simulink model "JT9D_Model_Dyn"  (Simulink 8.5)
settings: Solver=ode4  StartTime=0.0  StopTime=30  FixedStep=0.04  RelTol=1e-3
values from neighbouring files (symbols this model uses):
  MWS = setup_Inputs(MWS)    [JT9D_setup_everything_Dyn.m]    (also in JT9D_setup_everything_Lin.m; JT9D_setup_everything_PWLinGen.m; JT9D_setup_everything_SS.m)
undefined symbols (not defined in the file or in its folder): stripchar_TMATS
libraries: Lib_Turbo_Duct_TMATS x5, Lib_Turbo_Compressor_TMATS x3, Lib_Solve_OuterLoopIntegrator_TMATS x2, Lib_Turbo_Shaft_TMATS x2, Lib_Turbo_TurbineNPSS_TMATS x2, Lib_Turbo_Nozzle_TMATS x2, Lib_Cntrl_SimplePIcontroller_TMATS x1, Lib_Solve_IterNRSolverJC_TMATS x1, Lib_Turbo_Burner_TMATS x1, Lib_Turbo_Inlet_TMATS x1, Lib_Turbo_Splitter_TMATS x1
settings Model: Creator=jwchapm2  LastModifiedBy=jwchapm2
settings DataIOCC: SignalLoggingSaveFormat=Dataset
settings DebuggingCC: SolverPrmCheckMsg=warning  FcnCallInpInsideContextMsg=EnableAllAsError
settings GRTTargetCC: CombineOutputUpdateFcns=on  GRTInterface=off

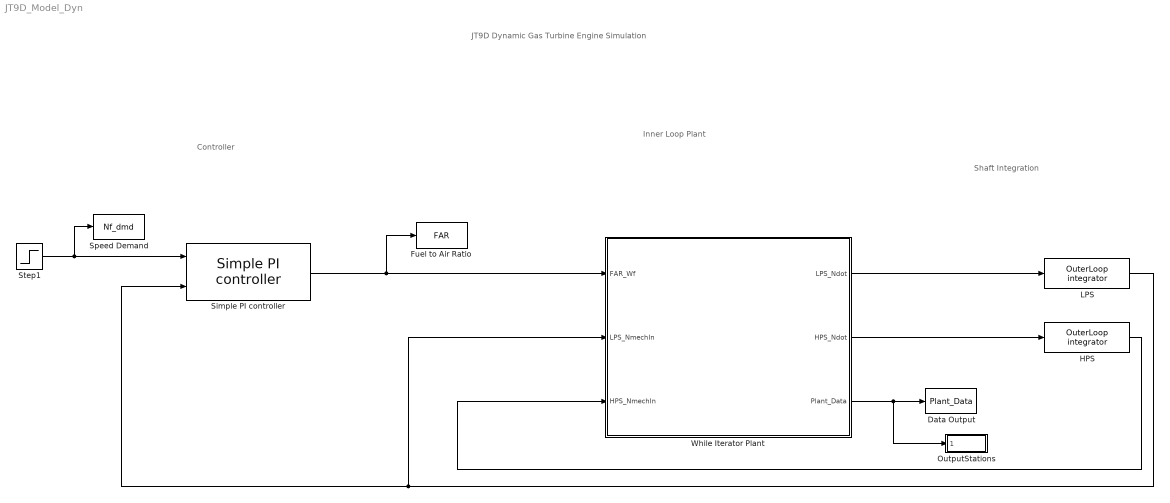
== system JT9D_Model_Dyn ==
  note: JT9D Dynamic Gas Turbine Engine Simulation
  note: Controller
  note: Inner Loop Plant
  note: Shaft Integration
  Data Output : ToWorkspace  VariableName=Plant_Data  SaveFormat=Timeseries  SampleTime=-1
  Fuel to Air Ratio : ToWorkspace  VariableName=FAR  SaveFormat=Timeseries  SampleTime=-1
  HPS : Lib_Solve_OuterLoopIntegrator_TMATS/OuterLoop integrator  OL_IC_M=MWS.Input.HP_Shaft
  LPS : Lib_Solve_OuterLoopIntegrator_TMATS/OuterLoop integrator  OL_IC_M=MWS.Input.LP_Shaft
  OutputStations : Subsystem
  Simple PI controller : Lib_Cntrl_SimplePIcontroller_TMATS/Simple PI controller  Kp_M=0.000008  Ki_M=0.00001  PI_IC_M=MWS.Input.FARin
  Speed Demand : ToWorkspace  VariableName=Nf_dmd  SaveFormat=Timeseries  SampleTime=-1
  Step1 : Step  Time=15  Before=MWS.Input.LP_Shaft  After=MWS.Input.LP_Shaft -200  SampleTime=0
  While Iterator Plant : Subsystem  TreatAsAtomicUnit=on
  wires:
  While Iterator Plant/1(LPS_Ndot) -> LPS/1
  While Iterator Plant/2(HPS_Ndot) -> HPS/1
  LPS/1 -> Simple PI controller/2, While Iterator Plant/2(LPS_NmechIn)
  HPS/1 -> While Iterator Plant/3(HPS_NmechIn)
  Simple PI controller/1 -> Fuel to Air Ratio/1, While Iterator Plant/1(FAR_Wf)
  Step1/1 -> Speed Demand/1, Simple PI controller/1
  While Iterator Plant/3(Plant_Data) -> OutputStations/1(DataBus), Data Output/1

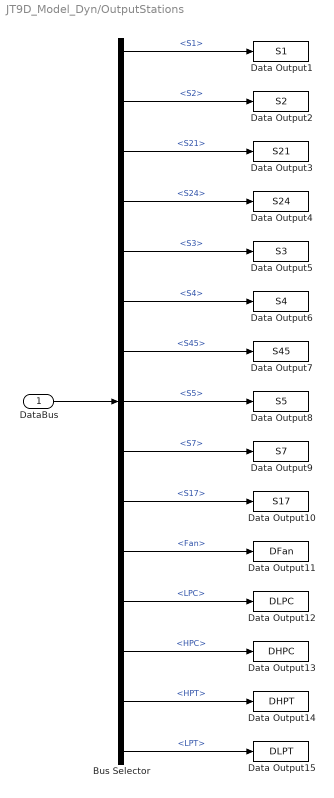
== system JT9D_Model_Dyn/OutputStations ==
  DataBus : Inport
  Bus Selector : BusSelector  OutputSignals=StationData.S1,StationData.S2,StationData.S21,StationData.S24,StationData.S3,StationData.S4,StationData.S45,StationData.S5,StationData.S7,StationData.S17,Data.Fan,Data.LPC,Data.HPC,Data.HPT,Data.LPT
  Data Output1 : ToWorkspace  VariableName=S1  SaveFormat=Timeseries  SampleTime=-1
  Data Output10 : ToWorkspace  VariableName=S17  SaveFormat=Timeseries  SampleTime=-1
  Data Output11 : ToWorkspace  VariableName=DFan  SaveFormat=Timeseries  SampleTime=-1
  Data Output12 : ToWorkspace  VariableName=DLPC  SaveFormat=Timeseries  SampleTime=-1
  Data Output13 : ToWorkspace  VariableName=DHPC  SaveFormat=Timeseries  SampleTime=-1
  Data Output14 : ToWorkspace  VariableName=DHPT  SaveFormat=Timeseries  SampleTime=-1
  Data Output15 : ToWorkspace  VariableName=DLPT  SaveFormat=Timeseries  SampleTime=-1
  Data Output2 : ToWorkspace  VariableName=S2  SaveFormat=Timeseries  SampleTime=-1
  Data Output3 : ToWorkspace  VariableName=S21  SaveFormat=Timeseries  SampleTime=-1
  Data Output4 : ToWorkspace  VariableName=S24  SaveFormat=Timeseries  SampleTime=-1
  Data Output5 : ToWorkspace  VariableName=S3  SaveFormat=Timeseries  SampleTime=-1
  Data Output6 : ToWorkspace  VariableName=S4  SaveFormat=Timeseries  SampleTime=-1
  Data Output7 : ToWorkspace  VariableName=S45  SaveFormat=Timeseries  SampleTime=-1
  Data Output8 : ToWorkspace  VariableName=S5  SaveFormat=Timeseries  SampleTime=-1
  Data Output9 : ToWorkspace  VariableName=S7  SaveFormat=Timeseries  SampleTime=-1
  wires:
  DataBus/1 -> Bus Selector/1
  Bus Selector/1 -> Data Output1/1  "<S1>"
  Bus Selector/2 -> Data Output2/1  "<S2>"
  Bus Selector/3 -> Data Output3/1  "<S21>"
  Bus Selector/4 -> Data Output4/1  "<S24>"
  Bus Selector/5 -> Data Output5/1  "<S3>"
  Bus Selector/6 -> Data Output6/1  "<S4>"
  Bus Selector/7 -> Data Output7/1  "<S45>"
  Bus Selector/8 -> Data Output8/1  "<S5>"
  Bus Selector/9 -> Data Output9/1  "<S7>"
  Bus Selector/10 -> Data Output10/1  "<S17>"
  Bus Selector/11 -> Data Output11/1  "<Fan>"
  Bus Selector/12 -> Data Output12/1  "<LPC>"
  Bus Selector/13 -> Data Output13/1  "<HPC>"
  Bus Selector/14 -> Data Output14/1  "<HPT>"
  Bus Selector/15 -> Data Output15/1  "<LPT>"

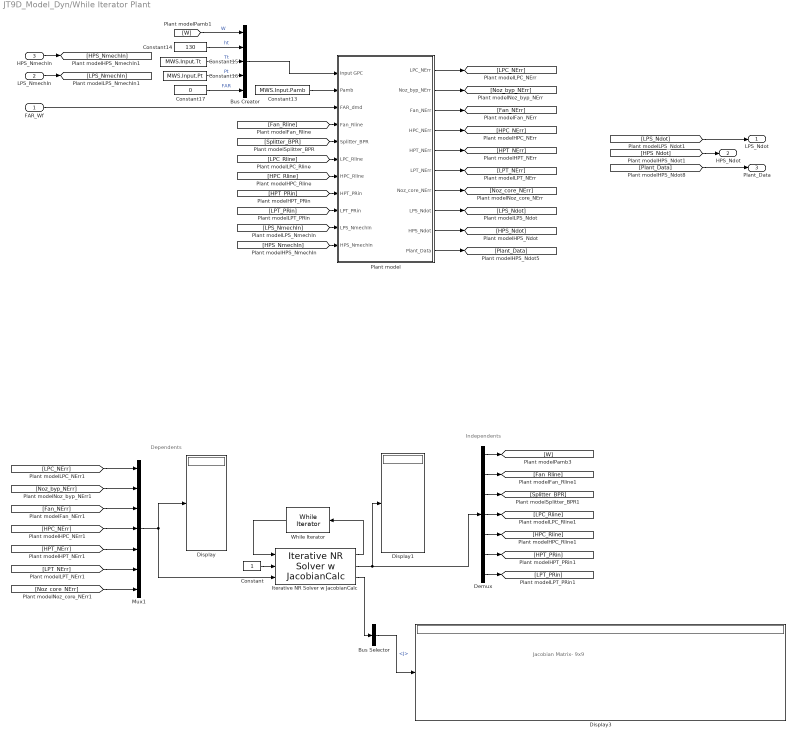
== system JT9D_Model_Dyn/While Iterator Plant ==
  note: Jacobian Matrix- 9x9
  note: Dependents
  note: Independents
  FAR_Wf : Inport
  LPS_NmechIn : Inport  Port=2
  HPS_NmechIn : Inport  Port=3
  Bus Creator : BusCreator  Inputs=5
  Bus Selector : BusSelector  OutputSignals=J
  Constant : Constant
  Constant13 : Constant  Value=MWS.Input.Pamb
  Constant14 : Constant  Value=130
  Constant15 : Constant  Value=MWS.Input.Tt
  Constant16 : Constant  Value=MWS.Input.Pt
  Constant17 : Constant  Value=0
  Demux : Demux  Outputs=7
  Display : Display
  Display1 : Display
  Display3 : Display
  Iterative NR Solver w JacobianCalc : Lib_Solve_IterNRSolverJC_TMATS/Iterative NR Solver w JacobianCalc  SJac_Per_M=[0.05 0.05 0.05 0.05 0.05 0.05 0.05]  SNR_IC_M=MWS.Input.NRICDyn  SNR_DX_M=5  SNR_Mx_M=100000  SNR_Mn_M=0.0001  SJacobianAttempts_M=20  Cond_Limits_M=0.0001
  Mux1 : Mux  Inputs=7
  Plant model : Subsystem
  While Iterator : WhileIterator  WhileBlockType=do-while  ShowIterationPort=on
  LPS_Ndot : Outport
  HPS_Ndot : Outport  Port=2
  Plant_Data : Outport  Port=3
  wires:
  [W] -> Bus Creator/1  "W"
  Bus Creator/1 -> Plant model/1(Input GPC)
  Constant17/1 -> Bus Creator/5  "FAR"
  Constant15/1 -> Bus Creator/3  "Tt"
  Constant16/1 -> Bus Creator/4  "Pt"
  Constant14/1 -> Bus Creator/2  "ht"
  Constant13/1 -> Plant model/2(Pamb)
  FAR_Wf/1 -> Plant model/3(FAR_dmd)
  [Fan_Rline] -> Plant model/4(Fan_Rline)
  [Splitter_BPR] -> Plant model/5(Splitter_BPR)
  [LPC_Rline] -> Plant model/6(LPC_Rline)
  [HPC_Rline] -> Plant model/7(HPC_Rline)
  [HPT_PRin] -> Plant model/8(HPT_PRin)
  [LPT_PRin] -> Plant model/9(LPT_PRin)
  [LPS_NmechIn] -> Plant model/10(LPS_NmechIn)
  [HPS_NmechIn] -> Plant model/11(HPS_NmechIn)
  Plant model/1(LPC_NErr) -> [LPC_NErr]
  Plant model/2(Noz_byp_NErr) -> [Noz_byp_NErr]
  Plant model/3(Fan_NErr) -> [Fan_NErr]
  Plant model/4(HPC_NErr) -> [HPC_NErr]
  Plant model/5(HPT_NErr) -> [HPT_NErr]
  Plant model/6(LPT_NErr) -> [LPT_NErr]
  Plant model/7(Noz_core_NErr) -> [Noz_core_NErr]
  Plant model/8(LPS_Ndot) -> [LPS_Ndot]
  Plant model/9(HPS_Ndot) -> [HPS_Ndot]
  Demux/1 -> [W]
  Demux/7 -> [LPT_PRin]
  Demux/5 -> [HPC_Rline]
  Demux/6 -> [HPT_PRin]
  Demux/4 -> [LPC_Rline]
  Demux/2 -> [Fan_Rline]
  Demux/3 -> [Splitter_BPR]
  [Fan_NErr] -> Mux1/3
  [HPC_NErr] -> Mux1/4
  [Noz_byp_NErr] -> Mux1/2
  [HPT_NErr] -> Mux1/5
  [LPC_NErr] -> Mux1/1
  [LPT_NErr] -> Mux1/6
  [Noz_core_NErr] -> Mux1/7
  Iterative NR Solver w JacobianCalc/3 -> Bus Selector/1
  Mux1/1 -> Iterative NR Solver w JacobianCalc/3, Display/1
  Bus Selector/1 -> Display3/1  "<J>"
  Iterative NR Solver w JacobianCalc/2 -> Demux/1, Display1/1
  Iterative NR Solver w JacobianCalc/1 -> While Iterator/1
  HPS_NmechIn/1 -> [HPS_NmechIn]
  LPS_NmechIn/1 -> [LPS_NmechIn]
  [LPS_Ndot] -> LPS_Ndot/1
  [HPS_Ndot] -> HPS_Ndot/1
  Plant model/10(Plant_Data) -> [Plant_Data]
  [Plant_Data] -> Plant_Data/1
  Constant/1 -> Iterative NR Solver w JacobianCalc/2
  While Iterator/1 -> Iterative NR Solver w JacobianCalc/1

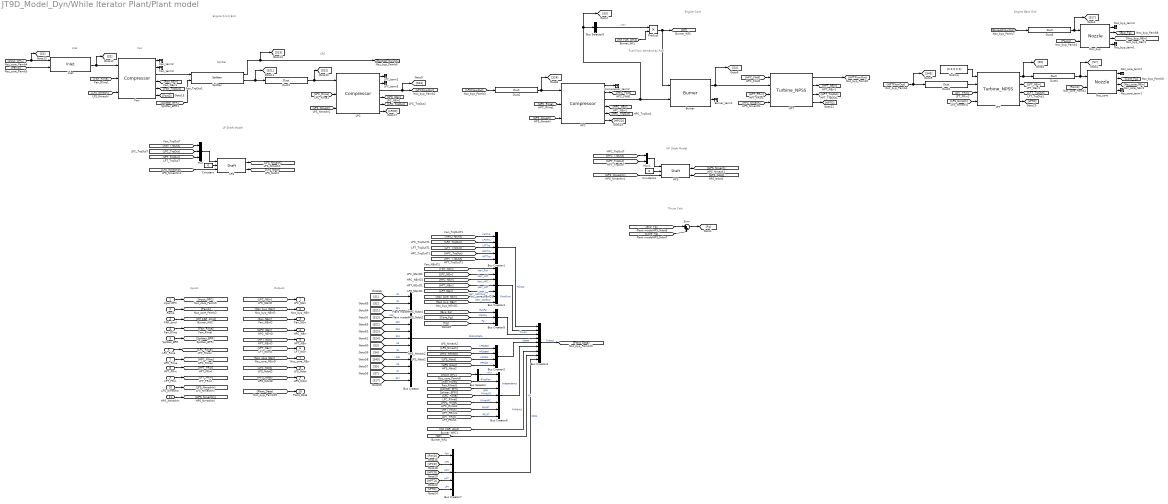
== system JT9D_Model_Dyn/While Iterator Plant/Plant model ==
  note: LP Shaft Model
  note: Inputs
  note: Outputs
  note: Engine Core
  note: HP Shaft Model
  note: Engine Back End
  note: Engine Front End
  note: Fuel Flow demand as FAR
  note: Inlet
  note: Fan
  note: Splitter
  note: LPC
  note: Thrust Calc
  Input GPC : Inport
  Pamb : Inport  Port=2
  FAR_dmd : Inport  Port=3
  Fan_Rline : Inport  Port=4
  Splitter_BPR : Inport  Port=5
  LPC_Rline : Inport  Port=6
  HPC_Rline : Inport  Port=7
  HPT_PRin : Inport  Port=8
  LPT_PRin : Inport  Port=9
  LPS_NmechIn : Inport  Port=10
  HPS_NmechIn : Inport  Port=11
  Burner : Lib_Turbo_Burner_TMATS/Burner  LHVEn_M=on  LHV_M=18400  Eff_M=0.994  hFuel_M=-1200  dPnormBurner_M=MWS.Burn.dP
  Burner_term1 : Terminator
  Bus Creator : BusCreator  Inputs=13
  Bus Creator1 : BusCreator  Inputs=5
  Bus Creator2 : BusCreator
  Bus Creator3 : BusCreator  Inputs=9
  Bus Creator4 : BusCreator  Inputs=7
  Bus Creator5 : BusCreator  Inputs=3
  Bus Creator6 : BusCreator  Inputs=7
  Bus Creator7 : BusCreator  Inputs=5
  Bus Selector : BusSelector  OutputSignals=W
  Bus Selector5 : BusSelector  OutputSignals=W
  Compressor_term2 : Terminator
  Constant : Constant  Value=0
  Constant1 : Constant  Value=0
  Duct1 : Lib_Turbo_Duct_TMATS/Duct  dP_M=MWS.Duct.dP1
  Duct2 : Lib_Turbo_Duct_TMATS/Duct  dP_M=MWS.Duct.dP2
  Duct3 : Lib_Turbo_Duct_TMATS/Duct  dP_M=MWS.Duct.dP3
  Duct4 : Lib_Turbo_Duct_TMATS/Duct  dP_M=MWS.Duct.dP4
  Duct5 : Lib_Turbo_Duct_TMATS/Duct  dP_M=MWS.Duct.dP5
  Fan : Lib_Turbo_Compressor_TMATS/Compressor  X_C_RlineVec_M=MWS.FAN.RlineVec  Z_C_AlphaVec_M=1  Y_C_Map_NcVec_M=MWS.FAN.NcVec  T_C_Map_WcArray_M=MWS.FAN.WcArray  T_C_Map_PRArray_M=MWS.FAN.PRArray  T_C_Map_EffArray_M=MWS.FAN.EffArray  s_C_Nc_M=MWS.FAN.s_Nc  s_C_Wc_M=MWS.FAN.s_Wc  s_C_PR_M=MWS.FAN.s_PR  s_C_Eff_M=MWS.FAN.s_eff  SL_M=off  Scale_M=none  CBLDEN_M=off  C_CBD_M=0  C_CBFht_M=0.5  C_CBFPt_M=0.5  FBLDEN_M=off  C_FBD_M=0  C_BFht_M=0.5  C_BFPt_M=0.5  DefSMEn_M=on  SRline_M=1  X_C_Map_WcSurgeVec_M=[0 200]  T_C_Map_PRSurgeVec_M=[30 30]  iDesign_M=MWS.iDes  NcDes_M=1  EffDes_M=0.8675  PRDes_M=1.645  RlineDes_M=2.3706  FVar_M=strcat('iDes_',stripchar_TMATS(gcb),'.bin')  BlkNm_M=double(gcb)  HP_M=off
  Fan_term2 : Terminator
  Fan_term3 : Terminator
  HPC : Lib_Turbo_Compressor_TMATS/Compressor  X_C_RlineVec_M=MWS.HPC.RlineVec  Z_C_AlphaVec_M=1  Y_C_Map_NcVec_M=MWS.HPC.NcVec  T_C_Map_WcArray_M=MWS.HPC.WcArray  T_C_Map_PRArray_M=MWS.HPC.PRArray  T_C_Map_EffArray_M=MWS.HPC.EffArray  s_C_Nc_M=MWS.HPC.s_Nc  s_C_Wc_M=MWS.HPC.s_Wc  s_C_PR_M=MWS.HPC.s_PR  s_C_Eff_M=MWS.HPC.s_eff  SL_M=off  Scale_M=none  CBLDEN_M=off  C_CBD_M=0  C_CBFht_M=0.5  C_CBFPt_M=0.5  FBLDEN_M=on  C_FBD_M=MWS.HPC.Fbld  C_BFht_M=MWS.HPC.Fblde  C_BFPt_M=MWS.HPC.Fbldp  DefSMEn_M=on  SRline_M=1  X_C_Map_WcSurgeVec_M=[0 200]  T_C_Map_PRSurgeVec_M=[30 30]  iDesign_M=MWS.iDes  NcDes_M=0.995  EffDes_M=.8651  PRDes_M=5.609  RlineDes_M=2.0424  FVar_M=strcat('iDes_',stripchar_TMATS(gcb),'.bin')  BlkNm_M=double(gcb)  HP_M=off
  HPS : Lib_Turbo_Shaft_TMATS/Shaft  Shaft_Inertia_M=MWS.Shaft.Iner_hp
  HPT : Lib_Turbo_TurbineNPSS_TMATS/Turbine_NPSS  X_T_Map_PRVec_M=MWS.HPT.PRVec  Y_T_Map_NcVec_M=MWS.HPT.NcVec  T_T_Map_WcArray_M=MWS.HPT.WcArray  T_T_Map_EffArray_M=MWS.HPT.EffArray  s_T_Nc_M=MWS.HPT.s_Nc  s_T_Wc_M=MWS.HPT.s_Wc  s_T_PR_M=MWS.HPT.s_PR  s_T_Eff_M=MWS.HPT.s_eff  ConfigNPSS_M=1  Scale_M=none  CFlwEn_M=on  T_CoolFlwPos_M=MWS.HPT.Cool  iDesign_M=MWS.iDes  NcDes_M=99.031  EffDes_M=.9133  PRDes_M=4.930  NDes_M=7390  FVar_M=strcat('iDes_',stripchar_TMATS(gcb),'.bin')  BlkNm_M=double(gcb)  HP_M=off
  Inlet : Lib_Turbo_Inlet_TMATS/Inlet  eRambase_M=MWS.Inlet.eRamBase  X_eRamVec_M=MWS.Inlet.eRamVec  T_eRamtbl_M=MWS.Inlet.eRamtbl
  LPC : Lib_Turbo_Compressor_TMATS/Compressor  X_C_RlineVec_M=MWS.LPC.RlineVec  Z_C_AlphaVec_M=1  Y_C_Map_NcVec_M=MWS.LPC.NcVec  T_C_Map_WcArray_M=MWS.LPC.WcArray  T_C_Map_PRArray_M=MWS.LPC.PRArray  T_C_Map_EffArray_M=MWS.LPC.EffArray  s_C_Nc_M=MWS.LPC.s_Nc  s_C_Wc_M=MWS.LPC.s_Wc  s_C_PR_M=MWS.LPC.s_PR  s_C_Eff_M=MWS.LPC.s_eff  SL_M=off  Scale_M=none  CBLDEN_M=off  C_CBD_M=0  C_CBFht_M=0.5  C_CBFPt_M=0.5  FBLDEN_M=off  C_FBD_M=0  C_BFht_M=0.5  C_BFPt_M=0.5  DefSMEn_M=on  SRline_M=1  X_C_Map_WcSurgeVec_M=[0 200]  T_C_Map_PRSurgeVec_M=[30 30]  iDesign_M=MWS.iDes  NcDes_M=0.993  EffDes_M=.8683  PRDes_M=2.488  RlineDes_M=1.7664  FVar_M=strcat('iDes_',stripchar_TMATS(gcb),'.bin')  BlkNm_M=double(gcb)  HP_M=off
  LPC_term2 : Terminator
  LPC_term3 : Terminator
  LPS : Lib_Turbo_Shaft_TMATS/Shaft  Shaft_Inertia_M=MWS.Shaft.Iner_lp
  LPT : Lib_Turbo_TurbineNPSS_TMATS/Turbine_NPSS  X_T_Map_PRVec_M=MWS.LPT.PRVec  Y_T_Map_NcVec_M=MWS.LPT.NcVec  T_T_Map_WcArray_M=MWS.LPT.WcArray  T_T_Map_EffArray_M=MWS.LPT.EffArray  s_T_Nc_M=MWS.LPT.s_Nc  s_T_Wc_M=MWS.LPT.s_Wc  s_T_PR_M=MWS.LPT.s_PR  s_T_Eff_M=MWS.LPT.s_eff  ConfigNPSS_M=1  Scale_M=none  CFlwEn_M=off  T_CoolFlwPos_M=0  iDesign_M=MWS.iDes  NcDes_M=105.038  EffDes_M=.9323  PRDes_M=6.420  NDes_M=3667.6  FVar_M=strcat('iDes_',stripchar_TMATS(gcb),'.bin')  BlkNm_M=double(gcb)  HP_M=off
  Mux : Mux  Inputs=3
  Mux1 : Mux  Inputs=2
  NoFlow : Constant  Value=[0 0 0 0 0]
  Noz_byp : Lib_Turbo_Nozzle_TMATS/Nozzle  SWType_M=Convergent  N_TArea_M=MWS.NozB.Ath  N_EArea_M=110.7  N_FL_M=0.00  X_N_TtVec2_M=[300 2000]  T_N_TGArray_M=[1 1]  X_N_PEQPaVec_M=[0 10000]  T_N_CdThArray_M=[1 1]  T_N_CvArray_M=MWS.NozB.CvArray  CfgEn_M=off  T_N_CfgArray_M=[1 1]  X_N_FARVec_M=[0; 0.0050; 0.0100; 0.0150; 0.0200; 0.0250; 0.0300]  T_N_RtArray_M="[0.0686;    0.0686;    0.0686;    0.0686;    0.0686;    0.0686;    0.0686]"  Y_N_TtVec_M=[300 2000]  T_N_MAP_gammaArray_M=[ 1.4 1.4 1.4 1.4 1.4 1.4 1.4; 1.4 1.4 1.4 1.4 1.4 1.4 1.4]  iDesign_M=MWS.iDes  WDes_M=562.61  FVar_M=strcat('iDes_',stripchar_TMATS(gcb),'.bin')
  Noz_byp_term1 : Terminator
  Noz_byp_term3 : Terminator
  Noz_core : Lib_Turbo_Nozzle_TMATS/Nozzle  SWType_M=Convergent  N_TArea_M=MWS.Noz.Ath  N_EArea_M=110.7  N_FL_M=0.00  X_N_TtVec2_M=[300 2000]  T_N_TGArray_M=[1 1]  X_N_PEQPaVec_M=[0 10000]  T_N_CdThArray_M=[1 1]  T_N_CvArray_M=MWS.Noz.CvArray  CfgEn_M=off  T_N_CfgArray_M=[1 1]  X_N_FARVec_M=[0; 0.0050; 0.0100; 0.0150; 0.0200; 0.0250; 0.0300]  T_N_RtArray_M="[0.0686;    0.0686;    0.0686;    0.0686;    0.0686;    0.0686;    0.0686]"  Y_N_TtVec_M=[300 2000]  T_N_MAP_gammaArray_M=[ 1.4 1.4 1.4 1.4 1.4 1.4 1.4; 1.4 1.4 1.4 1.4 1.4 1.4 1.4]  iDesign_M=MWS.iDes  WDes_M=113.51  FVar_M=strcat('iDes_',stripchar_TMATS(gcb),'.bin')
  Noz_core_term1 : Terminator
  Noz_core_term2 : Terminator
  Product : Product  RndMeth=Zero
  Splitter : Lib_Turbo_Splitter_TMATS/Splitter
  Sum : Sum  Inputs=|++
  LPC_NErr : Outport
  Noz_byp_NErr : Outport  Port=2
  Fan_NErr : Outport  Port=3
  HPC_NErr : Outport  Port=4
  HPT_NErr : Outport  Port=5
  LPT_NErr : Outport  Port=6
  Noz_core_NErr : Outport  Port=7
  LPS_Ndot : Outport  Port=8
  HPS_Ndot : Outport  Port=9
  Plant_Data : Outport  Port=10
  wires:
  Fan_Rline/1 -> [Fan_Rline]
  HPS_NmechIn/1 -> [HPS_NmechIn]
  HPC_Rline/1 -> [HPC_Rline]
  LPT_PRin/1 -> [LPT_PRin]
  FAR_dmd/1 -> [Wf_FAR_dmd]
  Splitter_BPR/1 -> [Splitter_BPR]
  LPC_Rline/1 -> [LPC_Rline]
  HPT_PRin/1 -> [HPT_PRin]
  LPS_NmechIn/1 -> [LPS_NmechIn]
  Duct1/1 -> [S22], LPC/1
  Duct4/1 -> [S7], Noz_core/1
  HPC/6 -> [HPCD]
  Noz_core/4 -> Noz_core_term1/1
  [Pamb] -> Noz_core/2
  Noz_core/3 -> [Noz_core_NErr]
  Duct3/1 -> LPT/2
  Noz_core/2 -> [Core_Fg]
  Mux/1 -> LPS/1
  Mux1/1 -> HPS/1
  [LPT_TrqOut] -> Mux/3
  [Fan_TrqOut] -> Mux/1
  [HPT_TrqOut] -> Mux1/2
  [HPC_TrqOut] -> Mux1/1
  [LPC_TrqOut] -> Mux/2
  HPS/2 -> [HPS_Ndot]
  HPS/1 -> [HPS_Nmech]
  [LPS_Nmech] -> Fan/3
  [LPS_Nmech] -> LPT/4
  [HPS_NmechIn] -> HPS/3
  [HPS_Nmech] -> HPC/3
  [LPS_Nmech] -> LPC/3
  Duct5/1 -> [S17], Noz_byp/1
  LPT/2 -> [LPT_NErr]
  [LPT_PRin] -> LPT/3
  [HPS_Nmech] -> HPT/4
  LPS/2 -> [LPS_Ndot]
  LPS/1 -> [LPS_Nmech]
  [LPS_NmechIn] -> LPS/3
  Splitter/2 -> [S21], Duct1/1
  Fan/3 -> Splitter/1
  Splitter/1 -> [S13], [BypassFlowOut]
  Burner/1 -> HPT/2, [S4]
  LPT/1 -> [S5], Duct4/1
  HPC/3 -> [S3], Bus Selector5/1, Burner/2
  LPC/3 -> [S23], [LPCFlowOut]
  HPT/2 -> [HPT_NErr]
  [HPT_PRin] -> HPT/3
  NoFlow/1 -> LPT/1
  Inlet/1 -> [S2], Fan/1
  LPT/3 -> [LPT_TrqOut]
  HPC/1 -> Compressor_term2/1
  Noz_byp/3 -> [Noz_byp_NErr]
  [Fan_Rline] -> Fan/2
  Noz_byp/1 -> Noz_byp_term3/1
  HPT/3 -> [HPT_TrqOut]
  Noz_byp/4 -> Noz_byp_term1/1
  [Pamb] -> Noz_byp/2
  Noz_byp/2 -> [Byp_Fg]
  Burner/2 -> Burner_term1/1
  LPC/2 -> LPC_term3/1
  LPC/4 -> [LPC_NErr]
  LPC/1 -> LPC_term2/1
  LPC/5 -> [LPC_TrqOut]
  [LPC_Rline] -> LPC/2
  [Splitter_BPR] -> Splitter/2
  [HPC_Fbld] -> HPT/1
  Fan/5 -> [Fan_TrqOut]
  Fan/4 -> [Fan_NErr]
  Fan/2 -> Fan_term3/1
  Fan/6 -> [FanD]
  Fan/1 -> Fan_term2/1
  HPC/5 -> [HPC_TrqOut]
  [HPC_Rline] -> HPC/2
  HPC/4 -> [HPC_NErr]
  HPC/2 -> [HPC_Fbld]
  LPC/6 -> [LPCD]
  [LPC_NErr] -> LPC_NErr/1
  [Noz_byp_NErr] -> Noz_byp_NErr/1
  [Fan_NErr] -> Fan_NErr/1
  [HPC_NErr] -> HPC_NErr/1
  [HPT_NErr] -> HPT_NErr/1
  [LPT_NErr] -> LPT_NErr/1
  [Noz_core_NErr] -> Noz_core_NErr/1
  [LPS_Ndot] -> LPS_Ndot/1
  [HPS_Ndot] -> HPS_Ndot/1
  [HPTFlowOut] -> [S45], Duct3/1
  [Wf_FAR_dmd] -> Product/2
  Bus Selector5/1 -> Product/1  "<W>"
  Product/1 -> [Wf], Burner/1
  Pamb/1 -> [Pamb]
  [Pamb] -> Inlet/2
  [Input_GPC] -> [S1], Inlet/1
  Input GPC/1 -> [Input_GPC]
  Noz_core/1 -> Noz_core_term2/1
  [LPCFlowOut] -> Duct2/1
  HPT/1 -> [HPTFlowOut]
  [BypassFlowOut] -> Duct5/1
  [Plant_Data] -> Plant_Data/1
  [S23] -> Bus Creator/6  "S23"
  [S22] -> Bus Creator/5  "S22"
  [S24] -> Bus Creator/7  "S24"
  [S3] -> Bus Creator/8  "S3"
  [S13] -> Bus Creator/4  "S13"
  [S4] -> Bus Creator/9  "S4"
  [S21] -> Bus Creator/3  "S21"
  [S45] -> Bus Creator/10  "S45"
  [S2] -> Bus Creator/2  "S2"
  [S1] -> Bus Creator/1  "S1"
  [S5] -> Bus Creator/11  "S5"
  [S7] -> Bus Creator/12  "S7"
  [S17] -> Bus Creator/13  "S17"
  Bus Creator/1 -> Bus Creator3/4  "StationData"
  Bus Creator2/1 -> Bus Creator3/5  "Speed"
  Bus Creator1/1 -> Bus Creator3/1  "Torque"
  Bus Creator3/1 -> [Plant_Data]  "Output"
  [Fan_NErr] -> Bus Creator4/1  "Nerr_Fan"
  [Noz_byp_NErr] -> Bus Creator4/7  "Nerr_NozByp"
  [LPC_NErr] -> Bus Creator4/2  "Nerr_LPC"
  [HPC_NErr] -> Bus Creator4/3  "Nerr_HPC"
  [HPT_NErr] -> Bus Creator4/4  "Nerr_HPT"
  [LPT_NErr] -> Bus Creator4/5  "Nerr_LPT"
  [Noz_core_NErr] -> Bus Creator4/6  "Nerr_NozCore"
  [Fan_TrqOut] -> Bus Creator1/1  "FanTrq"
  [LPC_TrqOut] -> Bus Creator1/2  "LPCTrq"
  [HPC_TrqOut] -> Bus Creator1/4  "HPCTrq"
  [HPT_TrqOut] -> Bus Creator1/5  "HPTTrq"
  [LPT_TrqOut] -> Bus Creator1/3  "LPTTrq"
  [Byp_Fg] -> Bus Creator5/1  "BypFg"
  [Core_Fg] -> Bus Creator5/2  "MainFg"
  [Fg] -> Bus Creator5/3  "Fg"
  [LPS_Nmech] -> Bus Creator2/1  "LPSpeed"
  [HPS_Nmech] -> Bus Creator2/2  "HPSpeed"
  [LPS_Ndot] -> Bus Creator2/3  "LPNdot"
  [HPS_Ndot] -> Bus Creator2/4  "HPNdot"
  [HPT_PRin] -> Bus Creator6/6  "PRHPT"
  [HPC_Rline] -> Bus Creator6/5  "RlineHPC"
  [Fan_Rline] -> Bus Creator6/2  "RlineFan"
  [Splitter_BPR] -> Bus Creator6/3  "BPR"
  [LPC_Rline] -> Bus Creator6/4  "RlineLPC"
  [LPT_PRin] -> Bus Creator6/7  "PRLPT"
  Bus Selector/1 -> Bus Creator6/1  "<W>"
  Bus Creator4/1 -> Bus Creator3/2  "FlowError"
  Bus Creator5/1 -> Bus Creator3/3  "Thrust"
  Bus Creator6/1 -> Bus Creator3/6  "Independents"
  [Wf_FAR_dmd] -> Bus Creator3/7  "FARdmd"
  [Byp_Fg] -> Sum/1
  [Core_Fg] -> Sum/2
  Sum/1 -> [Fg]
  Duct2/1 -> [S24], HPC/1
  [Wf] -> Bus Creator3/8  "Wf"
  [Input_GPC] -> Bus Selector/1
  HPT/4 -> [HPTD]
  LPT/4 -> [LPTD]
  [LPCD] -> Bus Creator7/2  "LPC"
  [FanD] -> Bus Creator7/1  "Fan"
  [HPCD] -> Bus Creator7/3  "HPC"
  [HPTD] -> Bus Creator7/4  "HPT"
  [LPTD] -> Bus Creator7/5  "LPT"
  Bus Creator7/1 -> Bus Creator3/9  "Data"
  Constant/1 -> LPS/2
  Constant1/1 -> HPS/2
